simulink model "NoV2GG2V"  (R2017a)
settings: Solver=ode23t  StartTime=0.0  StopTime=10  RelTol=1e-3
values from neighbouring files (symbols this model uses):
  C_Vdc = 100*18e-3    (= 1.8)    [main_v2gg2v.m]
  Cf = 10*165e-6    (= 0.00165)    [main_v2gg2v.m]
  D = 20    [main_v2gg2v.m]
  E1 = 1.07364213042869    (= 1.07364213043)    [main_v2gg2v.m]
  E2 = 1.05726676017896    (= 1.05726676018)    [main_v2gg2v.m]
  E3 = 1.05298913370226    (= 1.0529891337)    [main_v2gg2v.m]
  f_grid = 50    [main_v2gg2v.m]
  H1 = 10    [main_v2gg2v.m]
  H2 = 15    [main_v2gg2v.m]
  H3 = 60    [main_v2gg2v.m]
  h_PEV = -2000    [main_v2gg2v.m]
  Ibat_ref = -200    [main_v2gg2v.m]
  Ibatfault_ref = 200    [main_v2gg2v.m]
  Ki_CC = 1    [main_v2gg2v.m]
  Ki_inner = 5000    [main_v2gg2v.m]
  Ki_outer = 10000    [main_v2gg2v.m]
  Ki_PLL = 10000    [main_v2gg2v.m]
  Kp_CC = 10    [main_v2gg2v.m]
  Kp_inner = 100    [main_v2gg2v.m]
  Kp_outer = 250    [main_v2gg2v.m]
  Kp_PLL = 100    [main_v2gg2v.m]
  Lbat = 2e-3    (= 0.002)    [main_v2gg2v.m]
  Lgrid = 1/10*0.69e-3    (= 6.9e-05)    [main_v2gg2v.m]
  Linv = 1/10*0.48e-3    (= 4.8e-05)    [main_v2gg2v.m]
  LowSat_CC = 0    [main_v2gg2v.m]
  omega = 2*pi*f_grid    (= 314.159265359)    [main_v2gg2v.m]
  Pm1 = 2.49    [main_v2gg2v.m]
  Pm2 = 4.21    [main_v2gg2v.m]
  Pm3 = 8.20    (= 8.2)    [main_v2gg2v.m]
  Rd = 1.31    [main_v2gg2v.m]
  S1pu = (1.5 + .45j)    [main_v2gg2v.m]
  S2pu = (1.0 + .3j)    [main_v2gg2v.m]
  S3pu = (12.4 + 2.5j)    [main_v2gg2v.m]
  Sbase = 1e6    (= 1000000)    [main_v2gg2v.m]
  Snom_trafo = 1050e6    (= 1050000000)    [main_v2gg2v.m]
  t_fault_end = t_fault_start + FCT    (= 0.723)    [main_v2gg2v.m]
  t_fault_start = 0.5    [main_v2gg2v.m]
  Ts = 1e-5    (= 1e-05)    [main_v2gg2v.m]
  UpSat_CC = 1    [main_v2gg2v.m]
  Vbase = 345e3    (= 345000)    [main_v2gg2v.m]
  Vdc_ref = 1.5e3    (= 1500)    [main_v2gg2v.m]
  Vfault_thresh = 455    [main_v2gg2v.m]
undefined symbols (not defined in the file or in its folder): D1, Delta, Ion, L12, L13, L23, Lbuckboost, Lithium, R_Vdc, Rbuckboost
libraries: powerlib x175, powerlib_meascontrol x55, simulink x45, electricdrivelib x30, dspstat3 x3
(part 2 of 5)

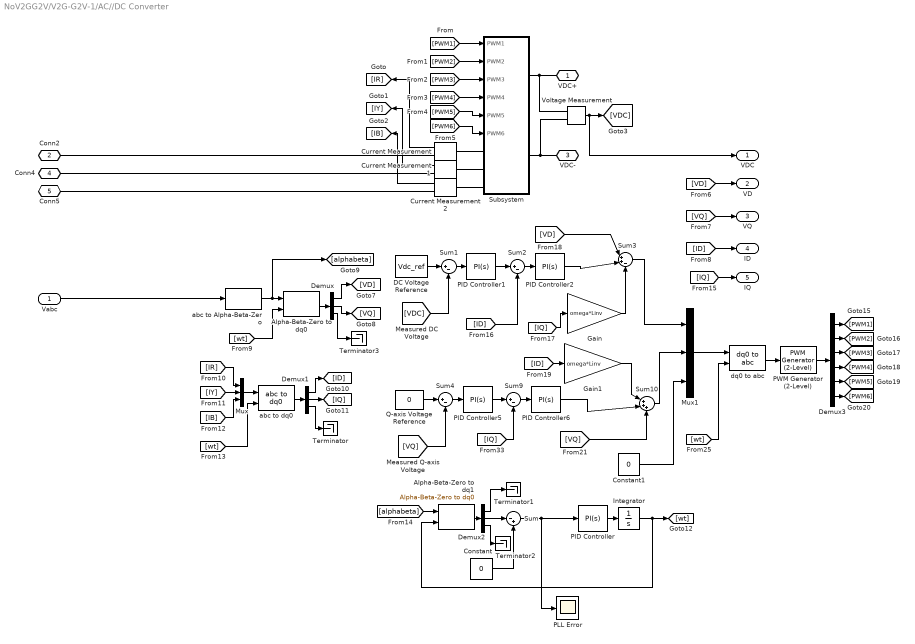
== system NoV2GG2V/V2G-G2V-1/AC//DC Converter ==
  Vabc : Inport
  Alpha-Beta-Zero to dq0 : powerlib_meascontrol/Transformations/Alpha-Beta-Zero to dq0  Alignment=90 degrees behind phase A axis
      settings: SourceProductName=Simscape Power Systems
  Alpha-Beta-Zero to dq1 : powerlib_meascontrol/Transformations/Alpha-Beta-Zero to dq0  Alignment=90 degrees behind phase A axis
      settings: SourceProductName=Simscape Power Systems
  Constant : Constant  Value=0
  Constant1 : Constant  Value=0
  Current Measurement : powerlib/Measurements/Current Measurement  PhasorSimulation=off  OutputType=Complex  PSBequivalent=0
  Current Measurement1 : powerlib/Measurements/Current Measurement  PhasorSimulation=off  OutputType=Complex  PSBequivalent=0
  Current Measurement2 : powerlib/Measurements/Current Measurement  PhasorSimulation=off  OutputType=Complex  PSBequivalent=0
  DC Voltage Reference : Constant  Value=Vdc_ref
  Demux : Demux  Outputs=3
  Demux1 : Demux  Outputs=3
  Demux2 : Demux  Outputs=3
  Demux3 : Demux  Outputs=6
  Gain : Gain  Gain=omega*Linv
  Gain1 : Gain  Gain=omega*Linv
  Integrator : Integrator
  Mux : Mux  Inputs=3
  Mux1 : Mux  Inputs=3
  PID Controller : simulink/Continuous/PID Controller  Controller=PI  TimeDomain=Continuous-time  SampleTime=-1  IntegratorMethod=Forward Euler  FilterMethod=Forward Euler  Form=Parallel  UseFilter=on  ControllerParametersSource=internal  P=Kp_PLL  I=Ki_PLL  D=0  N=100  InitialConditionSource=internal  InitialConditionForIntegrator=0  InitialConditionForFilter=0  ExternalReset=none  ZeroCross=off  LimitOutput=off  UpperSaturationLimit=inf  LowerSaturationLimit=-inf  LinearizeAsGain=on  AntiWindupMode=none  Kb=1  TrackingMode=off  Kt=1  PParamMin=[]  PParamMax=[]  IParamMin=[]  IParamMax=[]  DParamMin=[]  DParamMax=[]  NParamMin=[]  NParamMax=[]  KbParamMin=[]  KbParamMax=[]  KtParamMin=[]  KtParamMax=[]  POutMin=[]  POutMax=[]  IOutMin=[]  IOutMax=[]  DOutMin=[]  DOutMax=[]  NOutMin=[]  NOutMax=[]  KbOutMin=[]  KbOutMax=[]  KtOutMin=[]  KtOutMax=[]  IntegratorOutMin=[]  IntegratorOutMax=[]  FilterOutMin=[]  FilterOutMax=[]  SumOutMin=[]  SumOutMax=[]  SumI1OutMin=[]  SumI1OutMax=[]  SumI2OutMin=[]  SumI2OutMax=[]  SumI3OutMin=[]  SumI3OutMax=[]  SumDOutMin=[]  SumDOutMax=[]  SaturationOutMin=[]  SaturationOutMax=[]  IntegratorContinuousStateAttributes=''  IntegratorStateMustResolveToSignalObject=off  IntegratorRTWStateStorageClass=Auto  FilterContinuousStateAttributes=''  FilterStateMustResolveToSignalObject=off  FilterRTWStateStorageClass=Auto  DifferentiatorICPrevScaledInput=0  DifferentiatorOutMin=[]  DifferentiatorOutMax=[]  InitialConditionSetting=State (most efficient)
  PID Controller1 : simulink/Continuous/PID Controller  Controller=PI  TimeDomain=Continuous-time  SampleTime=-1  IntegratorMethod=Forward Euler  FilterMethod=Forward Euler  Form=Parallel  UseFilter=on  ControllerParametersSource=internal  P=Kp_outer  I=Ki_outer  D=0  N=100  InitialConditionSource=internal  InitialConditionForIntegrator=0  InitialConditionForFilter=0  ExternalReset=none  ZeroCross=off  LimitOutput=off  UpperSaturationLimit=inf  LowerSaturationLimit=-inf  LinearizeAsGain=on  AntiWindupMode=none  Kb=1  TrackingMode=off  Kt=1  PParamMin=[]  PParamMax=[]  IParamMin=[]  IParamMax=[]  DParamMin=[]  DParamMax=[]  NParamMin=[]  NParamMax=[]  KbParamMin=[]  KbParamMax=[]  KtParamMin=[]  KtParamMax=[]  POutMin=[]  POutMax=[]  IOutMin=[]  IOutMax=[]  DOutMin=[]  DOutMax=[]  NOutMin=[]  NOutMax=[]  KbOutMin=[]  KbOutMax=[]  KtOutMin=[]  KtOutMax=[]  IntegratorOutMin=[]  IntegratorOutMax=[]  FilterOutMin=[]  FilterOutMax=[]  SumOutMin=[]  SumOutMax=[]  SumI1OutMin=[]  SumI1OutMax=[]  SumI2OutMin=[]  SumI2OutMax=[]  SumI3OutMin=[]  SumI3OutMax=[]  SumDOutMin=[]  SumDOutMax=[]  SaturationOutMin=[]  SaturationOutMax=[]  IntegratorContinuousStateAttributes=''  IntegratorStateMustResolveToSignalObject=off  IntegratorRTWStateStorageClass=Auto  FilterContinuousStateAttributes=''  FilterStateMustResolveToSignalObject=off  FilterRTWStateStorageClass=Auto  DifferentiatorICPrevScaledInput=0  DifferentiatorOutMin=[]  DifferentiatorOutMax=[]  InitialConditionSetting=State (most efficient)
  PID Controller2 : simulink/Continuous/PID Controller  Controller=PI  TimeDomain=Continuous-time  SampleTime=-1  IntegratorMethod=Forward Euler  FilterMethod=Forward Euler  Form=Parallel  UseFilter=on  ControllerParametersSource=internal  P=Kp_inner  I=Ki_inner  D=0  N=100  InitialConditionSource=internal  InitialConditionForIntegrator=0  InitialConditionForFilter=0  ExternalReset=none  LimitOutput=off  UpperSaturationLimit=inf  LowerSaturationLimit=-inf  LinearizeAsGain=on  AntiWindupMode=none  Kb=1  TrackingMode=off  Kt=1  PParamMin=[]  PParamMax=[]  IParamMin=[]  IParamMax=[]  DParamMin=[]  DParamMax=[]  NParamMin=[]  NParamMax=[]  KbParamMin=[]  KbParamMax=[]  KtParamMin=[]  KtParamMax=[]  POutMin=[]  POutMax=[]  IOutMin=[]  IOutMax=[]  DOutMin=[]  DOutMax=[]  NOutMin=[]  NOutMax=[]  KbOutMin=[]  KbOutMax=[]  KtOutMin=[]  KtOutMax=[]  IntegratorOutMin=[]  IntegratorOutMax=[]  FilterOutMin=[]  FilterOutMax=[]  SumOutMin=[]  SumOutMax=[]  SumI1OutMin=[]  SumI1OutMax=[]  SumI2OutMin=[]  SumI2OutMax=[]  SumI3OutMin=[]  SumI3OutMax=[]  SumDOutMin=[]  SumDOutMax=[]  SaturationOutMin=[]  SaturationOutMax=[]  IntegratorContinuousStateAttributes=''  IntegratorStateMustResolveToSignalObject=off  IntegratorRTWStateStorageClass=Auto  FilterContinuousStateAttributes=''  FilterStateMustResolveToSignalObject=off  FilterRTWStateStorageClass=Auto  DifferentiatorICPrevScaledInput=0  DifferentiatorOutMin=[]  DifferentiatorOutMax=[]  InitialConditionSetting=State (most efficient)
  PID Controller5 : simulink/Continuous/PID Controller  Controller=PI  TimeDomain=Continuous-time  SampleTime=-1  IntegratorMethod=Forward Euler  FilterMethod=Forward Euler  Form=Parallel  UseFilter=on  ControllerParametersSource=internal  P=Kp_outer  I=Ki_outer  D=0  N=100  InitialConditionSource=internal  InitialConditionForIntegrator=0  InitialConditionForFilter=0  ExternalReset=none  ZeroCross=off  LimitOutput=off  UpperSaturationLimit=inf  LowerSaturationLimit=-inf  LinearizeAsGain=on  AntiWindupMode=none  Kb=1  TrackingMode=off  Kt=1  PParamMin=[]  PParamMax=[]  IParamMin=[]  IParamMax=[]  DParamMin=[]  DParamMax=[]  NParamMin=[]  NParamMax=[]  KbParamMin=[]  KbParamMax=[]  KtParamMin=[]  KtParamMax=[]  POutMin=[]  POutMax=[]  IOutMin=[]  IOutMax=[]  DOutMin=[]  DOutMax=[]  NOutMin=[]  NOutMax=[]  KbOutMin=[]  KbOutMax=[]  KtOutMin=[]  KtOutMax=[]  IntegratorOutMin=[]  IntegratorOutMax=[]  FilterOutMin=[]  FilterOutMax=[]  SumOutMin=[]  SumOutMax=[]  SumI1OutMin=[]  SumI1OutMax=[]  SumI2OutMin=[]  SumI2OutMax=[]  SumI3OutMin=[]  SumI3OutMax=[]  SumDOutMin=[]  SumDOutMax=[]  SaturationOutMin=[]  SaturationOutMax=[]  IntegratorContinuousStateAttributes=''  IntegratorStateMustResolveToSignalObject=off  IntegratorRTWStateStorageClass=Auto  FilterContinuousStateAttributes=''  FilterStateMustResolveToSignalObject=off  FilterRTWStateStorageClass=Auto  DifferentiatorICPrevScaledInput=0  DifferentiatorOutMin=[]  DifferentiatorOutMax=[]  InitialConditionSetting=State (most efficient)
  PID Controller6 : simulink/Continuous/PID Controller  Controller=PI  TimeDomain=Continuous-time  SampleTime=-1  IntegratorMethod=Forward Euler  FilterMethod=Forward Euler  Form=Parallel  UseFilter=on  ControllerParametersSource=internal  P=Kp_inner  I=Ki_inner  D=0  N=100  InitialConditionSource=internal  InitialConditionForIntegrator=0  InitialConditionForFilter=0  ExternalReset=none  LimitOutput=off  UpperSaturationLimit=inf  LowerSaturationLimit=-inf  LinearizeAsGain=on  AntiWindupMode=none  Kb=1  TrackingMode=off  Kt=1  PParamMin=[]  PParamMax=[]  IParamMin=[]  IParamMax=[]  DParamMin=[]  DParamMax=[]  NParamMin=[]  NParamMax=[]  KbParamMin=[]  KbParamMax=[]  KtParamMin=[]  KtParamMax=[]  POutMin=[]  POutMax=[]  IOutMin=[]  IOutMax=[]  DOutMin=[]  DOutMax=[]  NOutMin=[]  NOutMax=[]  KbOutMin=[]  KbOutMax=[]  KtOutMin=[]  KtOutMax=[]  IntegratorOutMin=[]  IntegratorOutMax=[]  FilterOutMin=[]  FilterOutMax=[]  SumOutMin=[]  SumOutMax=[]  SumI1OutMin=[]  SumI1OutMax=[]  SumI2OutMin=[]  SumI2OutMax=[]  SumI3OutMin=[]  SumI3OutMax=[]  SumDOutMin=[]  SumDOutMax=[]  SaturationOutMin=[]  SaturationOutMax=[]  IntegratorContinuousStateAttributes=''  IntegratorStateMustResolveToSignalObject=off  IntegratorRTWStateStorageClass=Auto  FilterContinuousStateAttributes=''  FilterStateMustResolveToSignalObject=off  FilterRTWStateStorageClass=Auto  DifferentiatorICPrevScaledInput=0  DifferentiatorOutMin=[]  DifferentiatorOutMax=[]  InitialConditionSetting=State (most efficient)
  PLL Error : Scope
  PWM Generator (2-Level) : powerlib_meascontrol/Pulse & Signal Generators/PWM Generator (2-Level)  ModulatorType=Three-phase bridge (6 pulses)  ModulatorMode=Unsynchronized  Fc=f_SW  Pc=90  nF=27  MinMax="[ -1  1 ]"  SamplingTechnique=Natural  ModulatingSignals=off  m=0.8  Freq=60  Phase=0  Ts=0  ShowCarrierOutport=off
      settings: SourceProductName=Simscape Power Systems
  Q-axis Voltage Reference : Constant  Value=0
  Subsystem : Subsystem
  Sum : Sum  Inputs=|-+
  Sum{1..2,4,9} (4 alike) : Sum  Inputs=|+-
  Sum10 : Sum  Inputs=|+++
  Sum3 : Sum  Inputs=|++-
  Terminator{,1..3} (4 alike) : Terminator
  Voltage Measurement : powerlib/Measurements/Voltage Measurement  PhasorSimulation=off  OutputType=Complex  PSBequivalent=0
  abc to Alpha-Beta-Zero : powerlib_meascontrol/Transformations/abc to Alpha-Beta-Zero
      settings: SourceProductName=Simscape Power Systems
  abc to dq0 : powerlib_meascontrol/Transformations/abc to dq0  Alignment=90 degrees behind phase A axis
  dq0 to abc : powerlib_meascontrol/Transformations/dq0 to abc  Alignment=90 degrees behind phase A axis
  VDC+ : PMIOPort  Port=1  Side=Right
  Conn2 : PMIOPort  Port=2  Side=Left
  VDC- : PMIOPort  Port=3  Side=Right
  Conn4 : PMIOPort  Port=4  Side=Left
  Conn5 : PMIOPort  Port=5  Side=Left
  VDC : Outport
  VD : Outport  Port=2
  VQ : Outport  Port=3
  ID : Outport  Port=4
  IQ : Outport  Port=5
  wires:
  Constant1/1 -> Mux1/3
  Current Measurement/1 -> [IR]
  [PWM1] -> Subsystem/1(PWM1)
  Current Measurement2/1 -> [IB]
  Current Measurement1/1 -> [IY]
  Alpha-Beta-Zero to dq0/1 -> Demux/1
  Demux1/2 -> [IQ]
  abc to dq0/1 -> Demux1/1
  [alphabeta] -> Alpha-Beta-Zero to dq1/1
  [wt] -> Alpha-Beta-Zero to dq0/2
  Demux1/1 -> [ID]
  [IB] -> Mux/3
  [PWM6] -> Subsystem/6(PWM6)
  [PWM4] -> Subsystem/4(PWM4)
  Vabc/1 -> abc to Alpha-Beta-Zero/1
  Demux/1 -> [VD]
  [IR] -> Mux/1
  Mux/1 -> abc to dq0/1
  [wt] -> abc to dq0/2
  [PWM5] -> Subsystem/5(PWM5)
  [PWM3] -> Subsystem/3(PWM3)
  abc to Alpha-Beta-Zero/1 -> [alphabeta], Alpha-Beta-Zero to dq0/1
  [PWM2] -> Subsystem/2(PWM2)
  Demux/2 -> [VQ]
  [IY] -> Mux/2
  Demux3/6 -> [PWM6]
  Sum2/1 -> PID Controller2/1
  [wt] -> dq0 to abc/2
  [VDC] -> Sum1/2
  PID Controller1/1 -> Sum2/1
  Demux3/1 -> [PWM1]
  Demux3/5 -> [PWM5]
  Mux1/1 -> dq0 to abc/1
  Constant/1 -> Sum/2
  Sum/1 -> PLL Error/1, PID Controller/1
  dq0 to abc/1 -> PWM Generator (2-Level)/1
  PID Controller/1 -> Integrator/1
  Integrator/1 -> [wt], Alpha-Beta-Zero to dq1/2
  Sum1/1 -> PID Controller1/1
  Demux3/4 -> [PWM4]
  DC Voltage Reference/1 -> Sum1/1
  Alpha-Beta-Zero to dq1/1 -> Demux2/1
  [ID] -> Sum2/2
  Demux3/3 -> [PWM3]
  Demux2/2 -> Sum/1
  [IQ] -> Gain/1
  PWM Generator (2-Level)/1 -> Demux3/1
  Demux3/2 -> [PWM2]
  [IQ] -> Sum9/2
  Demux/3 -> Terminator3/1
  [ID] -> Gain1/1
  PID Controller6/1 -> Sum10/2
  PID Controller5/1 -> Sum9/1
  Q-axis Voltage Reference/1 -> Sum4/1
  PID Controller2/1 -> Sum3/2
  Sum3/1 -> Mux1/1
  Demux1/3 -> Terminator/1
  Demux2/1 -> Terminator1/1
  Demux2/3 -> Terminator2/1
  Gain/1 -> Sum3/3
  Sum4/1 -> PID Controller5/1
  [VD] -> Sum3/1
  [VQ] -> Sum4/2
  Sum9/1 -> PID Controller6/1
  Sum10/1 -> Mux1/2
  [VQ] -> Sum10/3
  Gain1/1 -> Sum10/1
  Voltage Measurement/1 -> VDC/1, [VDC]
  [VQ] -> VQ/1
  [ID] -> ID/1
  [IQ] -> IQ/1
  [VD] -> VD/1
  connections:
  VDC+/RConn1 -- Voltage Measurement/LConn1 -- Subsystem/RConn1
  Current Measurement/LConn1 -- Subsystem/LConn1
  Current Measurement2/RConn1 -- Conn5/RConn1
  Current Measurement1/RConn1 -- Conn4/RConn1
  Subsystem/LConn2 -- Current Measurement1/LConn1
  Current Measurement/RConn1 -- Conn2/RConn1
  Current Measurement2/LConn1 -- Subsystem/LConn3
  VDC-/RConn1 -- Voltage Measurement/LConn2 -- Subsystem/RConn2

== system NoV2GG2V/V2G-G2V-1/MovingRMSFaultDetect1 ==
  Vabc : Inport
  Iabc : Inport  Port=2
  Add : Sum  Inputs=+++
  Clock1 : Clock
  Constant : Constant  Value=Vfault_thresh
  Constant1 : Constant  Value=Ibatfault_ref
  Data Store Memory : DataStoreMemory  DataStoreName=first_fault  ReadBeforeWriteMsg=warning  WriteAfterWriteMsg=warning  WriteAfterReadMsg=warning  InitialValue=false  ShowAdditionalParam=off  OutDataTypeStr=boolean
  Data Store Read : DataStoreRead  DataStoreName=first_fault
  Data Store Write : DataStoreWrite  DataStoreName=first_fault
  Demux : Demux  Outputs=3
  Gain2 : Gain  Gain=1/3
  MATLAB Function : MATLAB Function  TreatAsAtomicUnit=on
  Moving RMS : dspstat3/Moving RMS  Method=Sliding window  SpecifyWindowLength=on  WindowLength=1/(f_grid*Ts)  ForgettingFactor=0.9  SimulateUsing=Code generation
      settings: SourceProductName=DSP System Toolbox  SourceProductBaseCode=DS
  RMS Voltage : Scope  Commented=on
  grid_VI_1 : Scope  NumInputPorts=2
  Vrms : Outport
  Ibat_ref : Outport  Port=2
  wires:
  Constant1/1 -> MATLAB Function/4(Ibat_ref)
  Moving RMS/1 -> Demux/1
  Demux/1 -> Add/1
  Add/1 -> Gain2/1
  MATLAB Function/2(first_fault) -> Data Store Write/1
  Gain2/1 -> Vrms/1, RMS Voltage/1, MATLAB Function/2(v)
  MATLAB Function/1(y) -> Ibat_ref/1
  Vabc/1 -> Moving RMS/1, grid_VI_1/1
  Clock1/1 -> MATLAB Function/3(t)
  Demux/2 -> Add/2
  Demux/3 -> Add/3
  Iabc/1 -> grid_VI_1/2
  Data Store Read/1 -> MATLAB Function/1("first_fault ")
  Constant/1 -> MATLAB Function/5(Vfault_thresh)

== system NoV2GG2V/V2G-G2V-1/V2G_Gajduk ==
  Vabc : Inport
  f_grid : Inport  Port=2
  Gain4 : Gain  Gain=h_PEV
  PLL (3ph) : powerlib_meascontrol/PLL/PLL (3ph)  Fmin=49  Par_Init=[0, f_grid]  ParK=[180, 3200, 1]  TcD=1e-4  MaxRateChangeFreq=12  FilterCutOffFreq=25  Ts=Ts  AGC=on
  Saturation : Saturate  UpperLimit=0.1*abs(h_PEV)  LowerLimit=-0.1*abs(h_PEV)
  Sum3 : Sum  Inputs=|+-
  Terminator : Terminator
  delta_f : Outport
  Ibat_ref : Outport  Port=2
  wires:
  Sum3/1 -> Gain4/1, delta_f/1
  PLL (3ph)/2 -> Terminator/1
  Gain4/1 -> Saturation/1
  Saturation/1 -> Ibat_ref/1
  PLL (3ph)/1 -> Sum3/1
  Vabc/1 -> PLL (3ph)/1
  f_grid/1 -> Sum3/2

== system NoV2GG2V/V2G-G2V-2/5 Charging Stations ==
  Ibat_ref : Inport
  Charging Station1 : Subsystem
  Charging Station10 : Subsystem  Commented=on
  Charging Station2 : Subsystem
  Charging Station3 : Subsystem
  Charging Station4 : Subsystem
  Charging Station5 : Subsystem
  Charging Station6 : Subsystem  Commented=on
  Charging Station7 : Subsystem  Commented=on
  Charging Station8 : Subsystem  Commented=on
  Charging Station9 : Subsystem  Commented=on
  VDC+ : PMIOPort  Port=1  Side=Left
  VDC- : PMIOPort  Port=2  Side=Left
  to_workspace : Outport
  SOC : Outport  Port=2
  Current : Outport  Port=3
  Voltage : Outport  Port=4
  wires:
  Charging Station1/3(Current) -> Current/1
  Charging Station1/2(SOC) -> SOC/1
  Charging Station1/4(Voltage) -> Voltage/1
  Charging Station1/1(to_workspace) -> to_workspace/1
  Ibat_ref/1 -> Charging Station10/1(Ibat_ref), Charging Station9/1(Ibat_ref), Charging Station8/1(Ibat_ref), Charging Station7/1(Ibat_ref), Charging Station6/1(Ibat_ref), Charging Station5/1(Ibat_ref), Charging Station4/1(Ibat_ref), Charging Station3/1(Ibat_ref), Charging Station2/1(Ibat_ref), Charging Station1/1(Ibat_ref)
  connections:
  Charging Station9/LConn2 -- Charging Station10/LConn2 -- VDC-/RConn1 -- Charging Station1/LConn2 -- Charging Station2/LConn2 -- Charging Station3/LConn2 -- Charging Station4/LConn2 -- Charging Station5/LConn2 -- Charging Station6/LConn2 -- Charging Station7/LConn2 -- Charging Station8/LConn2
  Charging Station9/LConn1 -- Charging Station10/LConn1 -- Charging Station1/LConn1 -- VDC+/RConn1 -- Charging Station2/LConn1 -- Charging Station3/LConn1 -- Charging Station4/LConn1 -- Charging Station5/LConn1 -- Charging Station6/LConn1 -- Charging Station7/LConn1 -- Charging Station8/LConn1

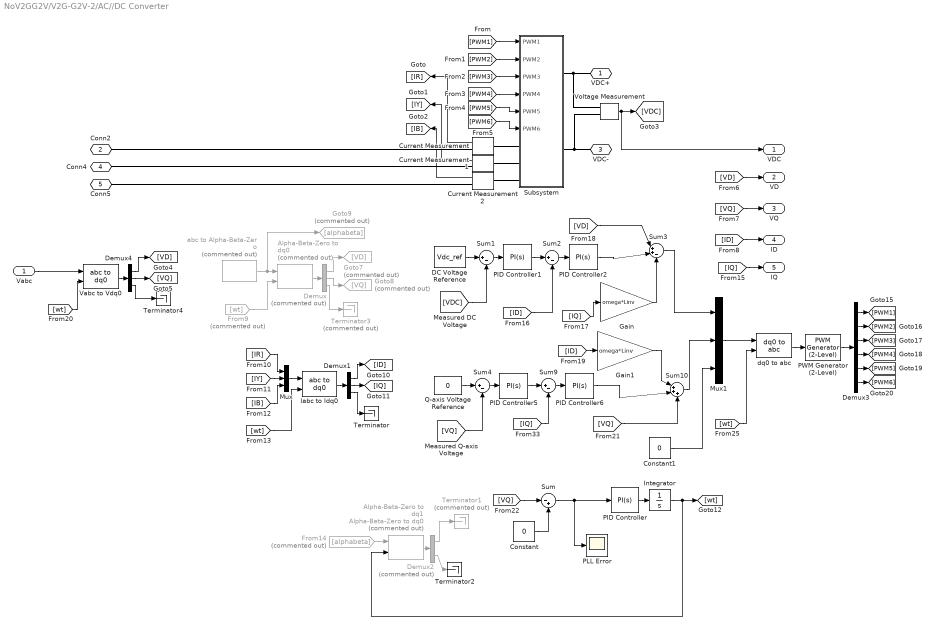
== system NoV2GG2V/V2G-G2V-2/AC//DC Converter ==
  Vabc : Inport
  Alpha-Beta-Zero to dq0 : powerlib_meascontrol/Transformations/Alpha-Beta-Zero to dq0  Commented=on  Alignment=90 degrees behind phase A axis
      settings: SourceProductName=Simscape Power Systems
  Alpha-Beta-Zero to dq1 : powerlib_meascontrol/Transformations/Alpha-Beta-Zero to dq0  Commented=on  Alignment=90 degrees behind phase A axis
      settings: SourceProductName=Simscape Power Systems
  Constant : Constant  Value=0
  Constant1 : Constant  Value=0
  Current Measurement : powerlib/Measurements/Current Measurement  PhasorSimulation=off  OutputType=Complex  PSBequivalent=0
  Current Measurement1 : powerlib/Measurements/Current Measurement  PhasorSimulation=off  OutputType=Complex  PSBequivalent=0
  Current Measurement2 : powerlib/Measurements/Current Measurement  PhasorSimulation=off  OutputType=Complex  PSBequivalent=0
  DC Voltage Reference : Constant  Value=Vdc_ref
  Demux : Demux  Commented=on  Outputs=3
  Demux1 : Demux  Outputs=3
  Demux2 : Demux  Commented=on  Outputs=3
  Demux3 : Demux  Outputs=6
  Demux4 : Demux  Outputs=3
  From14 : From  Commented=on  GotoTag=alphabeta
  From9 : From  Commented=on  GotoTag=wt
  Gain : Gain  Gain=omega*Linv
  Gain1 : Gain  Gain=omega*Linv
  Goto7 : Goto  Commented=on  GotoTag=VD
  Goto8 : Goto  Commented=on  GotoTag=VQ
  Goto9 : Goto  Commented=on  GotoTag=alphabeta
  Iabc to Idq0 : powerlib_meascontrol/Transformations/abc to dq0  Alignment=90 degrees behind phase A axis
  Integrator : Integrator
  Mux : Mux  Inputs=3
  Mux1 : Mux  Inputs=3
  PID Controller : simulink/Continuous/PID Controller  Controller=PI  TimeDomain=Continuous-time  SampleTime=-1  IntegratorMethod=Forward Euler  FilterMethod=Forward Euler  Form=Parallel  UseFilter=on  ControllerParametersSource=internal  P=Kp_PLL  I=Ki_PLL  D=0  N=100  InitialConditionSource=internal  InitialConditionForIntegrator=0  InitialConditionForFilter=0  ExternalReset=none  ZeroCross=off  LimitOutput=off  UpperSaturationLimit=inf  LowerSaturationLimit=-inf  LinearizeAsGain=on  AntiWindupMode=none  Kb=1  TrackingMode=off  Kt=1  PParamMin=[]  PParamMax=[]  IParamMin=[]  IParamMax=[]  DParamMin=[]  DParamMax=[]  NParamMin=[]  NParamMax=[]  KbParamMin=[]  KbParamMax=[]  KtParamMin=[]  KtParamMax=[]  POutMin=[]  POutMax=[]  IOutMin=[]  IOutMax=[]  DOutMin=[]  DOutMax=[]  NOutMin=[]  NOutMax=[]  KbOutMin=[]  KbOutMax=[]  KtOutMin=[]  KtOutMax=[]  IntegratorOutMin=[]  IntegratorOutMax=[]  FilterOutMin=[]  FilterOutMax=[]  SumOutMin=[]  SumOutMax=[]  SumI1OutMin=[]  SumI1OutMax=[]  SumI2OutMin=[]  SumI2OutMax=[]  SumI3OutMin=[]  SumI3OutMax=[]  SumDOutMin=[]  SumDOutMax=[]  SaturationOutMin=[]  SaturationOutMax=[]  IntegratorContinuousStateAttributes=''  IntegratorStateMustResolveToSignalObject=off  IntegratorRTWStateStorageClass=Auto  FilterContinuousStateAttributes=''  FilterStateMustResolveToSignalObject=off  FilterRTWStateStorageClass=Auto  DifferentiatorICPrevScaledInput=0  DifferentiatorOutMin=[]  DifferentiatorOutMax=[]  InitialConditionSetting=State (most efficient)
  PID Controller1 : simulink/Continuous/PID Controller  Controller=PI  TimeDomain=Continuous-time  SampleTime=-1  IntegratorMethod=Forward Euler  FilterMethod=Forward Euler  Form=Parallel  UseFilter=on  ControllerParametersSource=internal  P=Kp_outer  I=Ki_outer  D=0  N=100  InitialConditionSource=internal  InitialConditionForIntegrator=0  InitialConditionForFilter=0  ExternalReset=none  ZeroCross=off  LimitOutput=off  UpperSaturationLimit=inf  LowerSaturationLimit=-inf  LinearizeAsGain=on  AntiWindupMode=none  Kb=1  TrackingMode=off  Kt=1  PParamMin=[]  PParamMax=[]  IParamMin=[]  IParamMax=[]  DParamMin=[]  DParamMax=[]  NParamMin=[]  NParamMax=[]  KbParamMin=[]  KbParamMax=[]  KtParamMin=[]  KtParamMax=[]  POutMin=[]  POutMax=[]  IOutMin=[]  IOutMax=[]  DOutMin=[]  DOutMax=[]  NOutMin=[]  NOutMax=[]  KbOutMin=[]  KbOutMax=[]  KtOutMin=[]  KtOutMax=[]  IntegratorOutMin=[]  IntegratorOutMax=[]  FilterOutMin=[]  FilterOutMax=[]  SumOutMin=[]  SumOutMax=[]  SumI1OutMin=[]  SumI1OutMax=[]  SumI2OutMin=[]  SumI2OutMax=[]  SumI3OutMin=[]  SumI3OutMax=[]  SumDOutMin=[]  SumDOutMax=[]  SaturationOutMin=[]  SaturationOutMax=[]  IntegratorContinuousStateAttributes=''  IntegratorStateMustResolveToSignalObject=off  IntegratorRTWStateStorageClass=Auto  FilterContinuousStateAttributes=''  FilterStateMustResolveToSignalObject=off  FilterRTWStateStorageClass=Auto  DifferentiatorICPrevScaledInput=0  DifferentiatorOutMin=[]  DifferentiatorOutMax=[]  InitialConditionSetting=State (most efficient)
  PID Controller2 : simulink/Continuous/PID Controller  Controller=PI  TimeDomain=Continuous-time  SampleTime=-1  IntegratorMethod=Forward Euler  FilterMethod=Forward Euler  Form=Parallel  UseFilter=on  ControllerParametersSource=internal  P=Kp_inner  I=Ki_inner  D=0  N=100  InitialConditionSource=internal  InitialConditionForIntegrator=0  InitialConditionForFilter=0  ExternalReset=none  LimitOutput=off  UpperSaturationLimit=inf  LowerSaturationLimit=-inf  LinearizeAsGain=on  AntiWindupMode=none  Kb=1  TrackingMode=off  Kt=1  PParamMin=[]  PParamMax=[]  IParamMin=[]  IParamMax=[]  DParamMin=[]  DParamMax=[]  NParamMin=[]  NParamMax=[]  KbParamMin=[]  KbParamMax=[]  KtParamMin=[]  KtParamMax=[]  POutMin=[]  POutMax=[]  IOutMin=[]  IOutMax=[]  DOutMin=[]  DOutMax=[]  NOutMin=[]  NOutMax=[]  KbOutMin=[]  KbOutMax=[]  KtOutMin=[]  KtOutMax=[]  IntegratorOutMin=[]  IntegratorOutMax=[]  FilterOutMin=[]  FilterOutMax=[]  SumOutMin=[]  SumOutMax=[]  SumI1OutMin=[]  SumI1OutMax=[]  SumI2OutMin=[]  SumI2OutMax=[]  SumI3OutMin=[]  SumI3OutMax=[]  SumDOutMin=[]  SumDOutMax=[]  SaturationOutMin=[]  SaturationOutMax=[]  IntegratorContinuousStateAttributes=''  IntegratorStateMustResolveToSignalObject=off  IntegratorRTWStateStorageClass=Auto  FilterContinuousStateAttributes=''  FilterStateMustResolveToSignalObject=off  FilterRTWStateStorageClass=Auto  DifferentiatorICPrevScaledInput=0  DifferentiatorOutMin=[]  DifferentiatorOutMax=[]  InitialConditionSetting=State (most efficient)
  PID Controller5 : simulink/Continuous/PID Controller  Controller=PI  TimeDomain=Continuous-time  SampleTime=-1  IntegratorMethod=Forward Euler  FilterMethod=Forward Euler  Form=Parallel  UseFilter=on  ControllerParametersSource=internal  P=Kp_outer  I=Ki_outer  D=0  N=100  InitialConditionSource=internal  InitialConditionForIntegrator=0  InitialConditionForFilter=0  ExternalReset=none  ZeroCross=off  LimitOutput=off  UpperSaturationLimit=inf  LowerSaturationLimit=-inf  LinearizeAsGain=on  AntiWindupMode=none  Kb=1  TrackingMode=off  Kt=1  PParamMin=[]  PParamMax=[]  IParamMin=[]  IParamMax=[]  DParamMin=[]  DParamMax=[]  NParamMin=[]  NParamMax=[]  KbParamMin=[]  KbParamMax=[]  KtParamMin=[]  KtParamMax=[]  POutMin=[]  POutMax=[]  IOutMin=[]  IOutMax=[]  DOutMin=[]  DOutMax=[]  NOutMin=[]  NOutMax=[]  KbOutMin=[]  KbOutMax=[]  KtOutMin=[]  KtOutMax=[]  IntegratorOutMin=[]  IntegratorOutMax=[]  FilterOutMin=[]  FilterOutMax=[]  SumOutMin=[]  SumOutMax=[]  SumI1OutMin=[]  SumI1OutMax=[]  SumI2OutMin=[]  SumI2OutMax=[]  SumI3OutMin=[]  SumI3OutMax=[]  SumDOutMin=[]  SumDOutMax=[]  SaturationOutMin=[]  SaturationOutMax=[]  IntegratorContinuousStateAttributes=''  IntegratorStateMustResolveToSignalObject=off  IntegratorRTWStateStorageClass=Auto  FilterContinuousStateAttributes=''  FilterStateMustResolveToSignalObject=off  FilterRTWStateStorageClass=Auto  DifferentiatorICPrevScaledInput=0  DifferentiatorOutMin=[]  DifferentiatorOutMax=[]  InitialConditionSetting=State (most efficient)
  PID Controller6 : simulink/Continuous/PID Controller  Controller=PI  TimeDomain=Continuous-time  SampleTime=-1  IntegratorMethod=Forward Euler  FilterMethod=Forward Euler  Form=Parallel  UseFilter=on  ControllerParametersSource=internal  P=Kp_inner  I=Ki_inner  D=0  N=100  InitialConditionSource=internal  InitialConditionForIntegrator=0  InitialConditionForFilter=0  ExternalReset=none  LimitOutput=off  UpperSaturationLimit=inf  LowerSaturationLimit=-inf  LinearizeAsGain=on  AntiWindupMode=none  Kb=1  TrackingMode=off  Kt=1  PParamMin=[]  PParamMax=[]  IParamMin=[]  IParamMax=[]  DParamMin=[]  DParamMax=[]  NParamMin=[]  NParamMax=[]  KbParamMin=[]  KbParamMax=[]  KtParamMin=[]  KtParamMax=[]  POutMin=[]  POutMax=[]  IOutMin=[]  IOutMax=[]  DOutMin=[]  DOutMax=[]  NOutMin=[]  NOutMax=[]  KbOutMin=[]  KbOutMax=[]  KtOutMin=[]  KtOutMax=[]  IntegratorOutMin=[]  IntegratorOutMax=[]  FilterOutMin=[]  FilterOutMax=[]  SumOutMin=[]  SumOutMax=[]  SumI1OutMin=[]  SumI1OutMax=[]  SumI2OutMin=[]  SumI2OutMax=[]  SumI3OutMin=[]  SumI3OutMax=[]  SumDOutMin=[]  SumDOutMax=[]  SaturationOutMin=[]  SaturationOutMax=[]  IntegratorContinuousStateAttributes=''  IntegratorStateMustResolveToSignalObject=off  IntegratorRTWStateStorageClass=Auto  FilterContinuousStateAttributes=''  FilterStateMustResolveToSignalObject=off  FilterRTWStateStorageClass=Auto  DifferentiatorICPrevScaledInput=0  DifferentiatorOutMin=[]  DifferentiatorOutMax=[]  InitialConditionSetting=State (most efficient)
  PLL Error : Scope
  PWM Generator (2-Level) : powerlib_meascontrol/Pulse & Signal Generators/PWM Generator (2-Level)  ModulatorType=Three-phase bridge (6 pulses)  ModulatorMode=Unsynchronized  Fc=f_SW  Pc=90  nF=27  MinMax="[ -1  1 ]"  SamplingTechnique=Natural  ModulatingSignals=off  m=0.8  Freq=60  Phase=0  Ts=0  ShowCarrierOutport=off
      settings: SourceProductName=Simscape Power Systems
  Q-axis Voltage Reference : Constant  Value=0
  Subsystem : Subsystem
  Sum : Sum  Inputs=|-+
  Sum{1..2,4,9} (4 alike) : Sum  Inputs=|+-
  Sum10 : Sum  Inputs=|+++
  Sum3 : Sum  Inputs=|++-
  Terminator : Terminator
  Terminator1 : Terminator  Commented=on
  Terminator2 : Terminator
  Terminator3 : Terminator  Commented=on
  Terminator4 : Terminator
  Vabc to Vdq0 : powerlib_meascontrol/Transformations/abc to dq0  Alignment=90 degrees behind phase A axis
  Voltage Measurement : powerlib/Measurements/Voltage Measurement  PhasorSimulation=off  OutputType=Complex  PSBequivalent=0
  abc to Alpha-Beta-Zero : powerlib_meascontrol/Transformations/abc to Alpha-Beta-Zero  Commented=on
      settings: SourceProductName=Simscape Power Systems
  dq0 to abc : powerlib_meascontrol/Transformations/dq0 to abc  Alignment=90 degrees behind phase A axis
  VDC+ : PMIOPort  Port=1  Side=Right
  Conn2 : PMIOPort  Port=2  Side=Left
  VDC- : PMIOPort  Port=3  Side=Right
  Conn4 : PMIOPort  Port=4  Side=Left
  Conn5 : PMIOPort  Port=5  Side=Left
  VDC : Outport
  VD : Outport  Port=2
  VQ : Outport  Port=3
  ID : Outport  Port=4
  IQ : Outport  Port=5
  wires:
  Constant1/1 -> Mux1/3
  Current Measurement/1 -> [IR]
  [PWM1] -> Subsystem/1(PWM1)
  Current Measurement2/1 -> [IB]
  Current Measurement1/1 -> [IY]
  Alpha-Beta-Zero to dq0/1 -> Demux/1
  Demux1/2 -> [IQ]
  Iabc to Idq0/1 -> Demux1/1
  From14/1 -> Alpha-Beta-Zero to dq1/1
  From9/1 -> Alpha-Beta-Zero to dq0/2
  Demux1/1 -> [ID]
  [IB] -> Mux/3
  [PWM6] -> Subsystem/6(PWM6)
  [PWM4] -> Subsystem/4(PWM4)
  Demux/1 -> Goto7/1
  [IR] -> Mux/1
  Mux/1 -> Iabc to Idq0/1
  [wt] -> Iabc to Idq0/2
  [PWM5] -> Subsystem/5(PWM5)
  [PWM3] -> Subsystem/3(PWM3)
  abc to Alpha-Beta-Zero/1 -> Goto9/1, Alpha-Beta-Zero to dq0/1
  [PWM2] -> Subsystem/2(PWM2)
  Demux/2 -> Goto8/1
  [IY] -> Mux/2
  Demux3/6 -> [PWM6]
  Sum2/1 -> PID Controller2/1
  [wt] -> dq0 to abc/2
  [VDC] -> Sum1/2
  PID Controller1/1 -> Sum2/1
  Demux3/1 -> [PWM1]
  Demux3/5 -> [PWM5]
  Mux1/1 -> dq0 to abc/1
  Constant/1 -> Sum/2
  Sum/1 -> PLL Error/1, PID Controller/1
  dq0 to abc/1 -> PWM Generator (2-Level)/1
  PID Controller/1 -> Integrator/1
  Integrator/1 -> [wt], Alpha-Beta-Zero to dq1/2
  Sum1/1 -> PID Controller1/1
  Demux3/4 -> [PWM4]
  DC Voltage Reference/1 -> Sum1/1
  Alpha-Beta-Zero to dq1/1 -> Demux2/1
  [ID] -> Sum2/2
  Demux3/3 -> [PWM3]
  [IQ] -> Gain/1
  PWM Generator (2-Level)/1 -> Demux3/1
  Demux3/2 -> [PWM2]
  [IQ] -> Sum9/2
  Demux/3 -> Terminator3/1
  [ID] -> Gain1/1
  PID Controller6/1 -> Sum10/2
  PID Controller5/1 -> Sum9/1
  Q-axis Voltage Reference/1 -> Sum4/1
  PID Controller2/1 -> Sum3/2
  Sum3/1 -> Mux1/1
  Demux1/3 -> Terminator/1
  Demux2/1 -> Terminator1/1
  Demux2/3 -> Terminator2/1
  Gain/1 -> Sum3/3
  Sum4/1 -> PID Controller5/1
  [VD] -> Sum3/1
  [VQ] -> Sum4/2
  Sum9/1 -> PID Controller6/1
  Sum10/1 -> Mux1/2
  [VQ] -> Sum10/3
  Gain1/1 -> Sum10/1
  Voltage Measurement/1 -> VDC/1, [VDC]
  [VQ] -> VQ/1
  [ID] -> ID/1
  [IQ] -> IQ/1
  [VD] -> VD/1
  Vabc/1 -> Vabc to Vdq0/1
  Demux4/3 -> Terminator4/1
  Demux4/2 -> [VQ]
  Vabc to Vdq0/1 -> Demux4/1
  Demux4/1 -> [VD]
  [wt] -> Vabc to Vdq0/2
  [VQ] -> Sum/1
  connections:
  VDC+/RConn1 -- Voltage Measurement/LConn1 -- Subsystem/RConn1
  Current Measurement/LConn1 -- Subsystem/LConn1
  Current Measurement2/RConn1 -- Conn5/RConn1
  Current Measurement1/RConn1 -- Conn4/RConn1
  Subsystem/LConn2 -- Current Measurement1/LConn1
  Current Measurement/RConn1 -- Conn2/RConn1
  Current Measurement2/LConn1 -- Subsystem/LConn3
  VDC-/RConn1 -- Voltage Measurement/LConn2 -- Subsystem/RConn2

== system NoV2GG2V/V2G-G2V-2/MovingRMSFaultDetect2 ==
  Vabc : Inport
  Iabc : Inport  Port=2
  Add : Sum  Inputs=+++
  Clock1 : Clock
  Constant : Constant  Value=Vfault_thresh
  Constant1 : Constant  Value=Ibatfault_ref
  Data Store Memory : DataStoreMemory  DataStoreName=first_fault  ReadBeforeWriteMsg=warning  WriteAfterWriteMsg=warning  WriteAfterReadMsg=warning  InitialValue=false  ShowAdditionalParam=off  OutDataTypeStr=boolean
  Data Store Read : DataStoreRead  DataStoreName=first_fault
  Data Store Write : DataStoreWrite  DataStoreName=first_fault
  Demux : Demux  Outputs=3
  Gain2 : Gain  Gain=1/3
  MATLAB Function : MATLAB Function  TreatAsAtomicUnit=on
  Moving RMS : dspstat3/Moving RMS  Method=Sliding window  SpecifyWindowLength=on  WindowLength=1/(f_grid*Ts)  ForgettingFactor=0.9  SimulateUsing=Code generation
      settings: SourceProductName=DSP System Toolbox  SourceProductBaseCode=DS
  RMS Voltage : Scope  Commented=on
  grid_VI_2 : Scope  NumInputPorts=2
  Vrms : Outport
  Ibat_ref : Outport  Port=2
  wires:
  Constant1/1 -> MATLAB Function/4(Ibat_ref)
  Moving RMS/1 -> Demux/1
  Demux/1 -> Add/1
  Add/1 -> Gain2/1
  MATLAB Function/2(first_fault) -> Data Store Write/1
  Gain2/1 -> Vrms/1, RMS Voltage/1, MATLAB Function/2(v)
  MATLAB Function/1(y) -> Ibat_ref/1
  Vabc/1 -> Moving RMS/1, grid_VI_2/1
  Clock1/1 -> MATLAB Function/3(t)
  Demux/2 -> Add/2
  Demux/3 -> Add/3
  Iabc/1 -> grid_VI_2/2
  Data Store Read/1 -> MATLAB Function/1("first_fault ")
  Constant/1 -> MATLAB Function/5(Vfault_thresh)

== system NoV2GG2V/V2G-G2V-2/V2G_Gajduk ==
  Vabc : Inport
  f_grid : Inport  Port=2
  Gain4 : Gain  Gain=h_PEV
  PLL (3ph) : powerlib_meascontrol/PLL/PLL (3ph)  Fmin=49  Par_Init=[0, f_grid]  ParK=[180, 3200, 1]  TcD=1e-4  MaxRateChangeFreq=12  FilterCutOffFreq=25  Ts=Ts  AGC=on
  Saturation : Saturate  UpperLimit=0.1*abs(h_PEV)  LowerLimit=-0.1*abs(h_PEV)
  Sum3 : Sum  Inputs=|+-
  Terminator : Terminator
  delta_f : Outport
  Ibat_ref : Outport  Port=2
  wires:
  Sum3/1 -> Gain4/1, delta_f/1
  PLL (3ph)/2 -> Terminator/1
  Gain4/1 -> Saturation/1
  Saturation/1 -> Ibat_ref/1
  PLL (3ph)/1 -> Sum3/1
  Vabc/1 -> PLL (3ph)/1
  f_grid/1 -> Sum3/2

== system NoV2GG2V/V2G-G2V-3/5 Charging Stations ==
  Ibat_ref : Inport
  Charging Station1 : Subsystem
  Charging Station10 : Subsystem  Commented=on
  Charging Station2 : Subsystem
  Charging Station3 : Subsystem
  Charging Station4 : Subsystem
  Charging Station5 : Subsystem
  Charging Station6 : Subsystem  Commented=on
  Charging Station7 : Subsystem  Commented=on
  Charging Station8 : Subsystem  Commented=on
  Charging Station9 : Subsystem  Commented=on
  VDC+ : PMIOPort  Port=1  Side=Left
  VDC- : PMIOPort  Port=2  Side=Left
  to_workspace : Outport
  SOC : Outport  Port=2
  Current : Outport  Port=3
  Voltage : Outport  Port=4
  wires:
  Charging Station1/3(Current) -> Current/1
  Charging Station1/2(SOC) -> SOC/1
  Charging Station1/4(Voltage) -> Voltage/1
  Charging Station1/1(to_workspace) -> to_workspace/1
  Ibat_ref/1 -> Charging Station10/1(Ibat_ref), Charging Station9/1(Ibat_ref), Charging Station8/1(Ibat_ref), Charging Station7/1(Ibat_ref), Charging Station6/1(Ibat_ref), Charging Station5/1(Ibat_ref), Charging Station4/1(Ibat_ref), Charging Station3/1(Ibat_ref), Charging Station2/1(Ibat_ref), Charging Station1/1(Ibat_ref)
  connections:
  Charging Station9/LConn2 -- Charging Station10/LConn2 -- VDC-/RConn1 -- Charging Station1/LConn2 -- Charging Station2/LConn2 -- Charging Station3/LConn2 -- Charging Station4/LConn2 -- Charging Station5/LConn2 -- Charging Station6/LConn2 -- Charging Station7/LConn2 -- Charging Station8/LConn2
  Charging Station9/LConn1 -- Charging Station10/LConn1 -- Charging Station1/LConn1 -- VDC+/RConn1 -- Charging Station2/LConn1 -- Charging Station3/LConn1 -- Charging Station4/LConn1 -- Charging Station5/LConn1 -- Charging Station6/LConn1 -- Charging Station7/LConn1 -- Charging Station8/LConn1

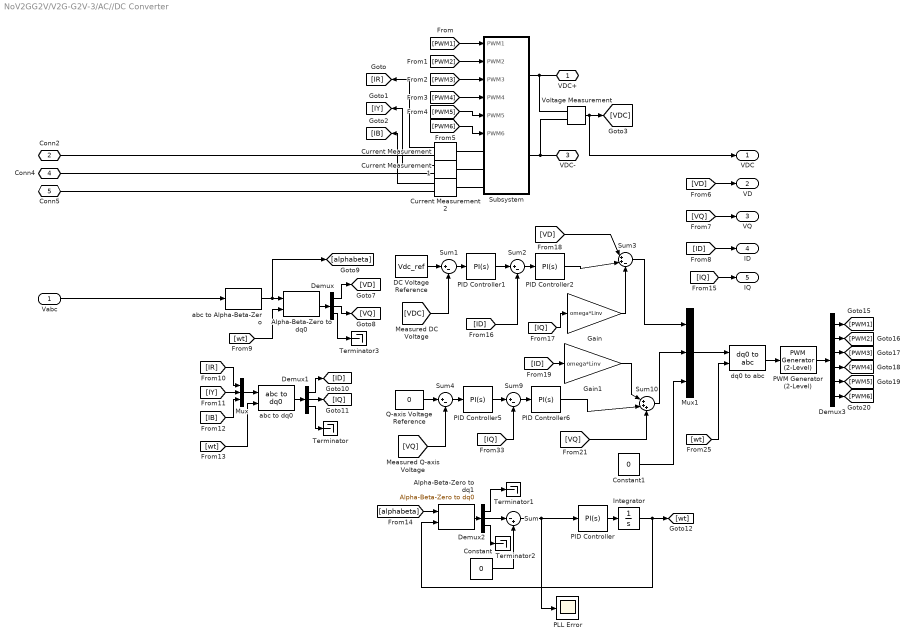
== system NoV2GG2V/V2G-G2V-3/AC//DC Converter ==
  Vabc : Inport
  Alpha-Beta-Zero to dq0 : powerlib_meascontrol/Transformations/Alpha-Beta-Zero to dq0  Alignment=90 degrees behind phase A axis
      settings: SourceProductName=Simscape Power Systems
  Alpha-Beta-Zero to dq1 : powerlib_meascontrol/Transformations/Alpha-Beta-Zero to dq0  Alignment=90 degrees behind phase A axis
      settings: SourceProductName=Simscape Power Systems
  Constant : Constant  Value=0
  Constant1 : Constant  Value=0
  Current Measurement : powerlib/Measurements/Current Measurement  PhasorSimulation=off  OutputType=Complex  PSBequivalent=0
  Current Measurement1 : powerlib/Measurements/Current Measurement  PhasorSimulation=off  OutputType=Complex  PSBequivalent=0
  Current Measurement2 : powerlib/Measurements/Current Measurement  PhasorSimulation=off  OutputType=Complex  PSBequivalent=0
  DC Voltage Reference : Constant  Value=Vdc_ref
  Demux : Demux  Outputs=3
  Demux1 : Demux  Outputs=3
  Demux2 : Demux  Outputs=3
  Demux3 : Demux  Outputs=6
  Gain : Gain  Gain=omega*Linv
  Gain1 : Gain  Gain=omega*Linv
  Integrator : Integrator
  Mux : Mux  Inputs=3
  Mux1 : Mux  Inputs=3
  PID Controller : simulink/Continuous/PID Controller  Controller=PI  TimeDomain=Continuous-time  SampleTime=-1  IntegratorMethod=Forward Euler  FilterMethod=Forward Euler  Form=Parallel  UseFilter=on  ControllerParametersSource=internal  P=Kp_PLL  I=Ki_PLL  D=0  N=100  InitialConditionSource=internal  InitialConditionForIntegrator=0  InitialConditionForFilter=0  ExternalReset=none  ZeroCross=off  LimitOutput=off  UpperSaturationLimit=inf  LowerSaturationLimit=-inf  LinearizeAsGain=on  AntiWindupMode=none  Kb=1  TrackingMode=off  Kt=1  PParamMin=[]  PParamMax=[]  IParamMin=[]  IParamMax=[]  DParamMin=[]  DParamMax=[]  NParamMin=[]  NParamMax=[]  KbParamMin=[]  KbParamMax=[]  KtParamMin=[]  KtParamMax=[]  POutMin=[]  POutMax=[]  IOutMin=[]  IOutMax=[]  DOutMin=[]  DOutMax=[]  NOutMin=[]  NOutMax=[]  KbOutMin=[]  KbOutMax=[]  KtOutMin=[]  KtOutMax=[]  IntegratorOutMin=[]  IntegratorOutMax=[]  FilterOutMin=[]  FilterOutMax=[]  SumOutMin=[]  SumOutMax=[]  SumI1OutMin=[]  SumI1OutMax=[]  SumI2OutMin=[]  SumI2OutMax=[]  SumI3OutMin=[]  SumI3OutMax=[]  SumDOutMin=[]  SumDOutMax=[]  SaturationOutMin=[]  SaturationOutMax=[]  IntegratorContinuousStateAttributes=''  IntegratorStateMustResolveToSignalObject=off  IntegratorRTWStateStorageClass=Auto  FilterContinuousStateAttributes=''  FilterStateMustResolveToSignalObject=off  FilterRTWStateStorageClass=Auto  DifferentiatorICPrevScaledInput=0  DifferentiatorOutMin=[]  DifferentiatorOutMax=[]  InitialConditionSetting=State (most efficient)
  PID Controller1 : simulink/Continuous/PID Controller  Controller=PI  TimeDomain=Continuous-time  SampleTime=-1  IntegratorMethod=Forward Euler  FilterMethod=Forward Euler  Form=Parallel  UseFilter=on  ControllerParametersSource=internal  P=Kp_outer  I=Ki_outer  D=0  N=100  InitialConditionSource=internal  InitialConditionForIntegrator=0  InitialConditionForFilter=0  ExternalReset=none  ZeroCross=off  LimitOutput=off  UpperSaturationLimit=inf  LowerSaturationLimit=-inf  LinearizeAsGain=on  AntiWindupMode=none  Kb=1  TrackingMode=off  Kt=1  PParamMin=[]  PParamMax=[]  IParamMin=[]  IParamMax=[]  DParamMin=[]  DParamMax=[]  NParamMin=[]  NParamMax=[]  KbParamMin=[]  KbParamMax=[]  KtParamMin=[]  KtParamMax=[]  POutMin=[]  POutMax=[]  IOutMin=[]  IOutMax=[]  DOutMin=[]  DOutMax=[]  NOutMin=[]  NOutMax=[]  KbOutMin=[]  KbOutMax=[]  KtOutMin=[]  KtOutMax=[]  IntegratorOutMin=[]  IntegratorOutMax=[]  FilterOutMin=[]  FilterOutMax=[]  SumOutMin=[]  SumOutMax=[]  SumI1OutMin=[]  SumI1OutMax=[]  SumI2OutMin=[]  SumI2OutMax=[]  SumI3OutMin=[]  SumI3OutMax=[]  SumDOutMin=[]  SumDOutMax=[]  SaturationOutMin=[]  SaturationOutMax=[]  IntegratorContinuousStateAttributes=''  IntegratorStateMustResolveToSignalObject=off  IntegratorRTWStateStorageClass=Auto  FilterContinuousStateAttributes=''  FilterStateMustResolveToSignalObject=off  FilterRTWStateStorageClass=Auto  DifferentiatorICPrevScaledInput=0  DifferentiatorOutMin=[]  DifferentiatorOutMax=[]  InitialConditionSetting=State (most efficient)
  PID Controller2 : simulink/Continuous/PID Controller  Controller=PI  TimeDomain=Continuous-time  SampleTime=-1  IntegratorMethod=Forward Euler  FilterMethod=Forward Euler  Form=Parallel  UseFilter=on  ControllerParametersSource=internal  P=Kp_inner  I=Ki_inner  D=0  N=100  InitialConditionSource=internal  InitialConditionForIntegrator=0  InitialConditionForFilter=0  ExternalReset=none  LimitOutput=off  UpperSaturationLimit=inf  LowerSaturationLimit=-inf  LinearizeAsGain=on  AntiWindupMode=none  Kb=1  TrackingMode=off  Kt=1  PParamMin=[]  PParamMax=[]  IParamMin=[]  IParamMax=[]  DParamMin=[]  DParamMax=[]  NParamMin=[]  NParamMax=[]  KbParamMin=[]  KbParamMax=[]  KtParamMin=[]  KtParamMax=[]  POutMin=[]  POutMax=[]  IOutMin=[]  IOutMax=[]  DOutMin=[]  DOutMax=[]  NOutMin=[]  NOutMax=[]  KbOutMin=[]  KbOutMax=[]  KtOutMin=[]  KtOutMax=[]  IntegratorOutMin=[]  IntegratorOutMax=[]  FilterOutMin=[]  FilterOutMax=[]  SumOutMin=[]  SumOutMax=[]  SumI1OutMin=[]  SumI1OutMax=[]  SumI2OutMin=[]  SumI2OutMax=[]  SumI3OutMin=[]  SumI3OutMax=[]  SumDOutMin=[]  SumDOutMax=[]  SaturationOutMin=[]  SaturationOutMax=[]  IntegratorContinuousStateAttributes=''  IntegratorStateMustResolveToSignalObject=off  IntegratorRTWStateStorageClass=Auto  FilterContinuousStateAttributes=''  FilterStateMustResolveToSignalObject=off  FilterRTWStateStorageClass=Auto  DifferentiatorICPrevScaledInput=0  DifferentiatorOutMin=[]  DifferentiatorOutMax=[]  InitialConditionSetting=State (most efficient)
  PID Controller5 : simulink/Continuous/PID Controller  Controller=PI  TimeDomain=Continuous-time  SampleTime=-1  IntegratorMethod=Forward Euler  FilterMethod=Forward Euler  Form=Parallel  UseFilter=on  ControllerParametersSource=internal  P=Kp_outer  I=Ki_outer  D=0  N=100  InitialConditionSource=internal  InitialConditionForIntegrator=0  InitialConditionForFilter=0  ExternalReset=none  ZeroCross=off  LimitOutput=off  UpperSaturationLimit=inf  LowerSaturationLimit=-inf  LinearizeAsGain=on  AntiWindupMode=none  Kb=1  TrackingMode=off  Kt=1  PParamMin=[]  PParamMax=[]  IParamMin=[]  IParamMax=[]  DParamMin=[]  DParamMax=[]  NParamMin=[]  NParamMax=[]  KbParamMin=[]  KbParamMax=[]  KtParamMin=[]  KtParamMax=[]  POutMin=[]  POutMax=[]  IOutMin=[]  IOutMax=[]  DOutMin=[]  DOutMax=[]  NOutMin=[]  NOutMax=[]  KbOutMin=[]  KbOutMax=[]  KtOutMin=[]  KtOutMax=[]  IntegratorOutMin=[]  IntegratorOutMax=[]  FilterOutMin=[]  FilterOutMax=[]  SumOutMin=[]  SumOutMax=[]  SumI1OutMin=[]  SumI1OutMax=[]  SumI2OutMin=[]  SumI2OutMax=[]  SumI3OutMin=[]  SumI3OutMax=[]  SumDOutMin=[]  SumDOutMax=[]  SaturationOutMin=[]  SaturationOutMax=[]  IntegratorContinuousStateAttributes=''  IntegratorStateMustResolveToSignalObject=off  IntegratorRTWStateStorageClass=Auto  FilterContinuousStateAttributes=''  FilterStateMustResolveToSignalObject=off  FilterRTWStateStorageClass=Auto  DifferentiatorICPrevScaledInput=0  DifferentiatorOutMin=[]  DifferentiatorOutMax=[]  InitialConditionSetting=State (most efficient)
  PID Controller6 : simulink/Continuous/PID Controller  Controller=PI  TimeDomain=Continuous-time  SampleTime=-1  IntegratorMethod=Forward Euler  FilterMethod=Forward Euler  Form=Parallel  UseFilter=on  ControllerParametersSource=internal  P=Kp_inner  I=Ki_inner  D=0  N=100  InitialConditionSource=internal  InitialConditionForIntegrator=0  InitialConditionForFilter=0  ExternalReset=none  LimitOutput=off  UpperSaturationLimit=inf  LowerSaturationLimit=-inf  LinearizeAsGain=on  AntiWindupMode=none  Kb=1  TrackingMode=off  Kt=1  PParamMin=[]  PParamMax=[]  IParamMin=[]  IParamMax=[]  DParamMin=[]  DParamMax=[]  NParamMin=[]  NParamMax=[]  KbParamMin=[]  KbParamMax=[]  KtParamMin=[]  KtParamMax=[]  POutMin=[]  POutMax=[]  IOutMin=[]  IOutMax=[]  DOutMin=[]  DOutMax=[]  NOutMin=[]  NOutMax=[]  KbOutMin=[]  KbOutMax=[]  KtOutMin=[]  KtOutMax=[]  IntegratorOutMin=[]  IntegratorOutMax=[]  FilterOutMin=[]  FilterOutMax=[]  SumOutMin=[]  SumOutMax=[]  SumI1OutMin=[]  SumI1OutMax=[]  SumI2OutMin=[]  SumI2OutMax=[]  SumI3OutMin=[]  SumI3OutMax=[]  SumDOutMin=[]  SumDOutMax=[]  SaturationOutMin=[]  SaturationOutMax=[]  IntegratorContinuousStateAttributes=''  IntegratorStateMustResolveToSignalObject=off  IntegratorRTWStateStorageClass=Auto  FilterContinuousStateAttributes=''  FilterStateMustResolveToSignalObject=off  FilterRTWStateStorageClass=Auto  DifferentiatorICPrevScaledInput=0  DifferentiatorOutMin=[]  DifferentiatorOutMax=[]  InitialConditionSetting=State (most efficient)
  PLL Error : Scope
  PWM Generator (2-Level) : powerlib_meascontrol/Pulse & Signal Generators/PWM Generator (2-Level)  ModulatorType=Three-phase bridge (6 pulses)  ModulatorMode=Unsynchronized  Fc=f_SW  Pc=90  nF=27  MinMax="[ -1  1 ]"  SamplingTechnique=Natural  ModulatingSignals=off  m=0.8  Freq=60  Phase=0  Ts=0  ShowCarrierOutport=off
      settings: SourceProductName=Simscape Power Systems
  Q-axis Voltage Reference : Constant  Value=0
  Subsystem : Subsystem
  Sum : Sum  Inputs=|-+
  Sum{1..2,4,9} (4 alike) : Sum  Inputs=|+-
  Sum10 : Sum  Inputs=|+++
  Sum3 : Sum  Inputs=|++-
  Terminator{,1..3} (4 alike) : Terminator
  Voltage Measurement : powerlib/Measurements/Voltage Measurement  PhasorSimulation=off  OutputType=Complex  PSBequivalent=0
  abc to Alpha-Beta-Zero : powerlib_meascontrol/Transformations/abc to Alpha-Beta-Zero
      settings: SourceProductName=Simscape Power Systems
  abc to dq0 : powerlib_meascontrol/Transformations/abc to dq0  Alignment=90 degrees behind phase A axis
  dq0 to abc : powerlib_meascontrol/Transformations/dq0 to abc  Alignment=90 degrees behind phase A axis
  VDC+ : PMIOPort  Port=1  Side=Right
  Conn2 : PMIOPort  Port=2  Side=Left
  VDC- : PMIOPort  Port=3  Side=Right
  Conn4 : PMIOPort  Port=4  Side=Left
  Conn5 : PMIOPort  Port=5  Side=Left
  VDC : Outport
  VD : Outport  Port=2
  VQ : Outport  Port=3
  ID : Outport  Port=4
  IQ : Outport  Port=5
  wires:
  Constant1/1 -> Mux1/3
  Current Measurement/1 -> [IR]
  [PWM1] -> Subsystem/1(PWM1)
  Current Measurement2/1 -> [IB]
  Current Measurement1/1 -> [IY]
  Alpha-Beta-Zero to dq0/1 -> Demux/1
  Demux1/2 -> [IQ]
  abc to dq0/1 -> Demux1/1
  [alphabeta] -> Alpha-Beta-Zero to dq1/1
  [wt] -> Alpha-Beta-Zero to dq0/2
  Demux1/1 -> [ID]
  [IB] -> Mux/3
  [PWM6] -> Subsystem/6(PWM6)
  [PWM4] -> Subsystem/4(PWM4)
  Vabc/1 -> abc to Alpha-Beta-Zero/1
  Demux/1 -> [VD]
  [IR] -> Mux/1
  Mux/1 -> abc to dq0/1
  [wt] -> abc to dq0/2
  [PWM5] -> Subsystem/5(PWM5)
  [PWM3] -> Subsystem/3(PWM3)
  abc to Alpha-Beta-Zero/1 -> [alphabeta], Alpha-Beta-Zero to dq0/1
  [PWM2] -> Subsystem/2(PWM2)
  Demux/2 -> [VQ]
  [IY] -> Mux/2
  Demux3/6 -> [PWM6]
  Sum2/1 -> PID Controller2/1
  [wt] -> dq0 to abc/2
  [VDC] -> Sum1/2
  PID Controller1/1 -> Sum2/1
  Demux3/1 -> [PWM1]
  Demux3/5 -> [PWM5]
  Mux1/1 -> dq0 to abc/1
  Constant/1 -> Sum/2
  Sum/1 -> PLL Error/1, PID Controller/1
  dq0 to abc/1 -> PWM Generator (2-Level)/1
  PID Controller/1 -> Integrator/1
  Integrator/1 -> [wt], Alpha-Beta-Zero to dq1/2
  Sum1/1 -> PID Controller1/1
  Demux3/4 -> [PWM4]
  DC Voltage Reference/1 -> Sum1/1
  Alpha-Beta-Zero to dq1/1 -> Demux2/1
  [ID] -> Sum2/2
  Demux3/3 -> [PWM3]
  Demux2/2 -> Sum/1
  [IQ] -> Gain/1
  PWM Generator (2-Level)/1 -> Demux3/1
  Demux3/2 -> [PWM2]
  [IQ] -> Sum9/2
  Demux/3 -> Terminator3/1
  [ID] -> Gain1/1
  PID Controller6/1 -> Sum10/2
  PID Controller5/1 -> Sum9/1
  Q-axis Voltage Reference/1 -> Sum4/1
  PID Controller2/1 -> Sum3/2
  Sum3/1 -> Mux1/1
  Demux1/3 -> Terminator/1
  Demux2/1 -> Terminator1/1
  Demux2/3 -> Terminator2/1
  Gain/1 -> Sum3/3
  Sum4/1 -> PID Controller5/1
  [VD] -> Sum3/1
  [VQ] -> Sum4/2
  Sum9/1 -> PID Controller6/1
  Sum10/1 -> Mux1/2
  [VQ] -> Sum10/3
  Gain1/1 -> Sum10/1
  Voltage Measurement/1 -> VDC/1, [VDC]
  [VQ] -> VQ/1
  [ID] -> ID/1
  [IQ] -> IQ/1
  [VD] -> VD/1
  connections:
  VDC+/RConn1 -- Voltage Measurement/LConn1 -- Subsystem/RConn1
  Current Measurement/LConn1 -- Subsystem/LConn1
  Current Measurement2/RConn1 -- Conn5/RConn1
  Current Measurement1/RConn1 -- Conn4/RConn1
  Subsystem/LConn2 -- Current Measurement1/LConn1
  Current Measurement/RConn1 -- Conn2/RConn1
  Current Measurement2/LConn1 -- Subsystem/LConn3
  VDC-/RConn1 -- Voltage Measurement/LConn2 -- Subsystem/RConn2

== system NoV2GG2V/V2G-G2V-3/MovingRMSFaultDetect2 ==
  Vabc : Inport
  Iabc : Inport  Port=2
  Add : Sum  Inputs=+++
  Clock1 : Clock
  Constant : Constant  Value=Vfault_thresh
  Constant1 : Constant  Value=Ibatfault_ref
  Data Store Memory : DataStoreMemory  DataStoreName=first_fault  ReadBeforeWriteMsg=warning  WriteAfterWriteMsg=warning  WriteAfterReadMsg=warning  InitialValue=false  ShowAdditionalParam=off  OutDataTypeStr=boolean
  Data Store Read : DataStoreRead  DataStoreName=first_fault
  Data Store Write : DataStoreWrite  DataStoreName=first_fault
  Demux : Demux  Outputs=3
  Gain2 : Gain  Gain=1/3
  MATLAB Function : MATLAB Function  TreatAsAtomicUnit=on
  Moving RMS : dspstat3/Moving RMS  Method=Sliding window  SpecifyWindowLength=on  WindowLength=1/(f_grid*Ts)  ForgettingFactor=0.9  SimulateUsing=Code generation
      settings: SourceProductName=DSP System Toolbox  SourceProductBaseCode=DS
  RMS Voltage : Scope  Commented=on
  grid_VI_2 : Scope  NumInputPorts=2
  Vrms : Outport
  Ibat_ref : Outport  Port=2
  wires:
  Constant1/1 -> MATLAB Function/4(Ibat_ref)
  Moving RMS/1 -> Demux/1
  Demux/1 -> Add/1
  Add/1 -> Gain2/1
  MATLAB Function/2(first_fault) -> Data Store Write/1
  Gain2/1 -> Vrms/1, RMS Voltage/1, MATLAB Function/2(v)
  MATLAB Function/1(y) -> Ibat_ref/1
  Vabc/1 -> Moving RMS/1, grid_VI_2/1
  Clock1/1 -> MATLAB Function/3(t)
  Demux/2 -> Add/2
  Demux/3 -> Add/3
  Iabc/1 -> grid_VI_2/2
  Data Store Read/1 -> MATLAB Function/1("first_fault ")
  Constant/1 -> MATLAB Function/5(Vfault_thresh)
